simulink model "a1bc1"  (R2020a)
settings: Solver=ode15s  StartTime=0.0  StopTime=10  RelTol=1e-3
undefined symbols (not defined in the file or in its folder): lamda
settings Model: Creator=mumun  LastModifiedBy=mumun

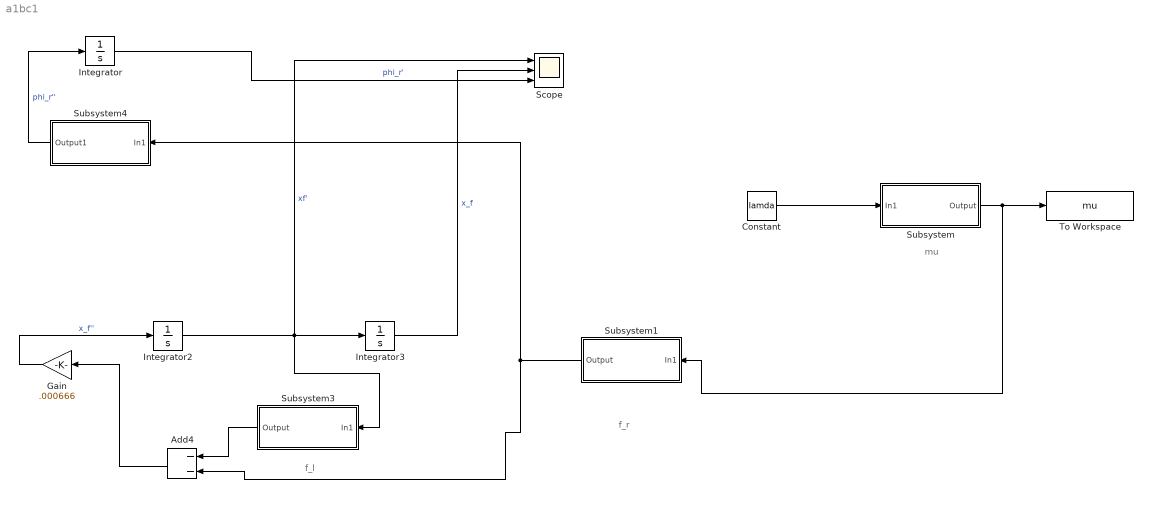
== system a1bc1 ==
  note: f_l
  note: f_r
  note: mu
  Add4 : Sum  Inputs=--
  Constant : Constant  Value=lamda
  Gain : Gain  Gain=.000666
  Integrator : Integrator  LimitOutput=on  LowerSaturationLimit=0
  Integrator2 : Integrator  InitialCondition=30  LimitOutput=on  LowerSaturationLimit=0
  Integrator3 : Integrator
  Scope : Scope  NumInputPorts=3
  Subsystem : Subsystem
  Subsystem1 : Subsystem
  Subsystem3 : Subsystem
  Subsystem4 : Subsystem
  To Workspace : ToWorkspace  VariableName=mu  SampleTime=-1
  wires:
  Integrator/1 -> Scope/3  "phi_r'"
  Integrator2/1 -> Scope/1, Subsystem3/1(In1), Integrator3/1  "xf'"
  Gain/1 -> Integrator2/1  "x_f''"
  Add4/1 -> Gain/1
  Subsystem1/1(Output) -> Subsystem4/1(In1), Add4/2
  Subsystem3/1(Output) -> Add4/1
  Subsystem4/1(Output1) -> Integrator/1  "phi_r''"
  Integrator3/1 -> Scope/2  "x_f"
  Constant/1 -> Subsystem/1(In1)
  Subsystem/1(Output) -> To Workspace/1, Subsystem1/1(In1)

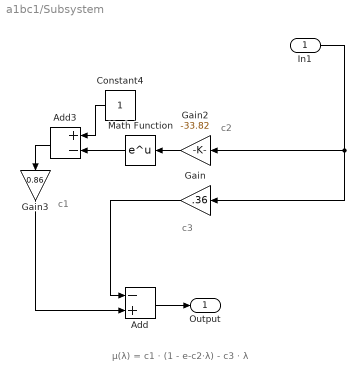
== system a1bc1/Subsystem ==
  note: c1
  note: c3
  note: c2
  note: µ(λ) = c1 · (1 - e-c2·λ) - c3 · λ
  In1 : Inport
  Add : Sum  Inputs=-+
  Add3 : Sum  Inputs=+-
  Constant4 : Constant
  Gain : Gain  Gain=.36
  Gain2 : Gain  Gain=-33.82
  Gain3 : Gain  Gain=0.86
  Math Function : Math  SaturateOnIntegerOverflow=on
  Output : Outport
  wires:
  Add3/1 -> Gain3/1
  Math Function/1 -> Add3/2
  Constant4/1 -> Add3/1
  Gain2/1 -> Math Function/1
  In1/1 -> Gain/1, Gain2/1
  Gain/1 -> Add/1
  Gain3/1 -> Add/2
  Add/1 -> Output/1

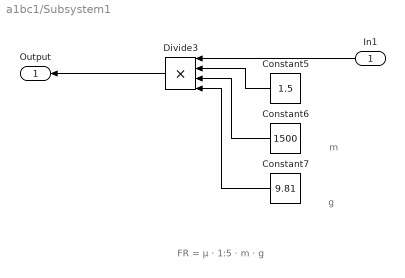
== system a1bc1/Subsystem1 ==
  note: m
  note: g
  note: FR = µ · 1:5 · m · g
  In1 : Inport
  Constant5 : Constant  Value=1.5
  Constant6 : Constant  Value=1500
  Constant7 : Constant  Value=9.81
  Divide3 : Product  Inputs=****
  Output : Outport
  wires:
  Constant6/1 -> Divide3/3
  In1/1 -> Divide3/1
  Constant5/1 -> Divide3/2
  Constant7/1 -> Divide3/4
  Divide3/1 -> Output/1

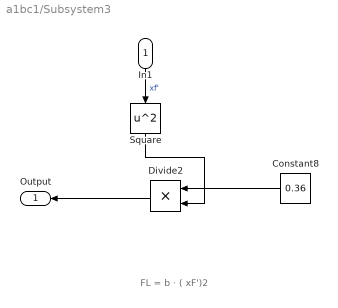
== system a1bc1/Subsystem3 ==
  note: FL = b · ( xF')2
  In1 : Inport
  Constant8 : Constant  Value=0.36
  Divide2 : Product  Inputs=**
  Square : Math  Operator=square  SaturateOnIntegerOverflow=on
  Output : Outport
  wires:
  In1/1 -> Square/1  "xf'"
  Divide2/1 -> Output/1
  Square/1 -> Divide2/2
  Constant8/1 -> Divide2/1

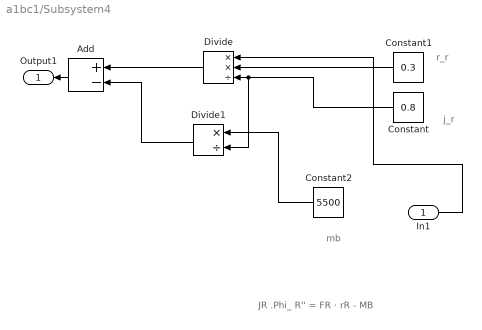
== system a1bc1/Subsystem4 ==
  note: JR .Phi_ R'' = FR · rR - MB
  note: mb
  note: r_r
  note: j_r
  In1 : Inport
  Add : Sum  Inputs=+-
  Constant : Constant  Value=0.8
  Constant1 : Constant  Value=0.3
  Constant2 : Constant  Value=5500
  Divide : Product  Inputs=**/
  Divide1 : Product  Inputs=*/
  Output1 : Outport
  wires:
  Divide/1 -> Add/1
  Divide1/1 -> Add/2
  Constant/1 -> Divide1/2, Divide/3
  Constant2/1 -> Divide1/1
  Constant1/1 -> Divide/2
  Add/1 -> Output1/1
  In1/1 -> Divide/1
